simulink model "EE405L_Lab3"  (R2021b)
settings: Solver=VariableStepAuto  StartTime=0.0  StopTime=30  RelTol=1e-3
settings Model: Creator=Kevin  LastModifiedBy=Kevin

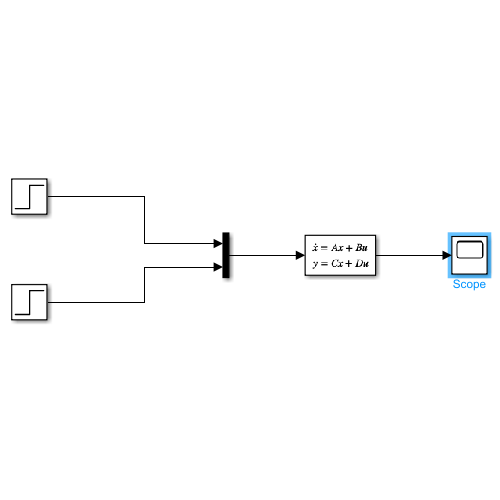
[thumbnail: Simulink's stored preview of the top-level diagram]
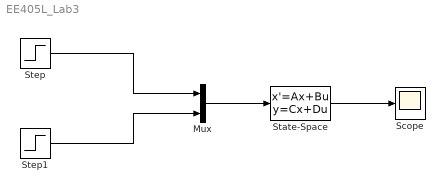
== system EE405L_Lab3 ==
  Mux : Mux  Inputs=2
  Scope : Scope
  State-Space : StateSpace  A=[-0.5572 -0.7814; 0.7814 0]  B=[1 -1; 0 2]  C=[1.9691 6.4493]  D=[0 0]  InitialCondition=[1; 0]
  Step : Step  SampleTime=0
  Step1 : Step  SampleTime=0
  wires:
  State-Space/1 -> Scope/1
  Mux/1 -> State-Space/1
  Step1/1 -> Mux/2
  Step/1 -> Mux/1
